simulink model "SOCPIControlBenchmark"  (R2021a)
settings: Solver=FixedStepAuto  StartTime=0.0  StopTime=tsim  FixedStep=0.01  RelTol=1e-3
values from neighbouring files (symbols this model uses):
  ET_Armature_Inductance_RO = 1.2298e-11    [benchmarkPIDStartRealDT.m]
  kio = 0.1    [benchmarkPIDStartRealDT.m]
  kpo = 0.3    [benchmarkPIDStartRealDT.m]
  M_Rotor_Inertia_RO = 1.8747e-13    [benchmarkPIDStartRealDT.m]
  maxKi = 0.3    [benchmarkPIDStartRealDT.m]
  maxKp = 0.5    [benchmarkPIDStartRealDT.m]
  minKi = 0.1    [benchmarkPIDStartRealDT.m]
  minKp = 0.1    [benchmarkPIDStartRealDT.m]
  N = 100    [benchmarkPIDStartRealDT.m]
  optimPeriod = 50    [benchmarkPIDStartRealDT.m]
  OVLim = 2    [benchmarkPIDStartRealDT.m]
  refSignalPeriod = optimPeriod    (= 50)    [benchmarkPIDStartRealDT.m]
  resetThreshold = 0.1    [benchmarkPIDStartRealDT.m]
  TSLim = 6    [benchmarkPIDStartRealDT.m]
libraries: fl_lib x11, nesl_utility x11, ee_lib x8, dspmathops x3, pid_lib x2, simulink x1
(part 2 of 4)

== matlab function SOCPIControlBenchmark/Original NM/Original NM Control/Original NM ==
  data: f input; y output size=2; x input; NM_state_val output
function [y, NM_state_val] = fcn(f, x)
% Acknowledgement goes to Mathworks' FMINSEARCH, borrowed some code snippets
% persistent count

persistent NM_state         %Integer definition for states, since enum is not supported
persistent Full_eval_count
persistent usual_delta      %5 percent deltas for non-zero terms
persistent zero_term_delta  %Even smaller delta for zero elements of x
persistent v fv v_r v_e v_m f_r v_c

n = 2;      %Input dimension - needs to be defined as a constant to keep Simulink port width inheretence happy
np1 = n+1;

n_r = 1/n;  %Calculate reciprocal at compilation time for mean calculation

%Simplex update coefficients %Can be a function of dimension see Han2010
alpha = 1;
beta = 2;
gamma = 0.5;
delta = 0.5;

%Adaptive simplex search coefficients: Han2010
% alpha = 1;
% beta = 1 + 2*n_r;
% gamma = 0.75 - 0.5*n_r;
% delta = 1 - n_r;
% 
% alpha = 0.25;
% beta = 1 + 2*n_r;
% gamma = 0.75 - 0.5*n_r;
% delta = 1 - n_r;


%NM_state:  
    %0 - Initial   (Initialize vertices)+++++
    %1 - FVE: Full vertex evaluation (with insertion sort after each
    %evaluation)++++++
    %2 - Insertion Sort (After Reflection, Expansion or Contraction Steps)
    %3 - Reflection Entry
    %4 - Reflection Evaluate+++++++++++++++++
    %5 - Expansion++++++++++++
    %6 - Outside Contraction++++++++++++
    %7 - Inside Contraction++++++++++++++++
    %(8) - Shrink (Implicit on contraction outcome)

%Full_eval_count:
    %Number of initial vertices evaluated


xin = x(:);         %Force xin to be a column vector

    if isempty(NM_state)
        v = zeros(n,np1);   %Initialize n+1 vertices for simplex
        fv = zeros(1,np1);  %function values at the vertices
        fv(1)=f;%initialize in the initial condition the first vertex
        
        
        v_m = v(:,1);       %0 vector centroid
        v_r = v_m;          %0 vector reflection   
        v_e = v_m;          %0 vector expansion
        v_c = v_m;          %0 vector contraction
        f_r = 0;          %0 vector

        usual_delta = 0.05;
        zero_term_delta = 0.00025;
        NM_state = 0;          %Initial state
        Full_eval_count = 1;   %No vertices evaulated, yet

        v(:,1) = xin;
        for j=1:n
            vt = xin;
            if vt(j) ~= 0
                vt(j) = (1 + usual_delta)*vt(j);
            else
                vt(j) = zero_term_delta;
            end
            v(:, j+1) = vt;
        end
        v;
    end
           
    switch NM_state  
        case 0 %Vertices has just been initialized
          y = v(:, Full_eval_count); %Write out first vertex for evaluation
          NM_state = 1;
          
        case 1 %Full vertex evaluation  and reflection on the final part
            fv(Full_eval_count) = f;  %Read evaluated function value
            
            %sort values
            j = Full_eval_count;  %New value came in, insert it into sorted list
            while ( (j>1) && (fv(j-1)>fv(j)) ) %Sort ascending
               temp = fv(j-1);
               fv(j-1) = fv(j);
               fv(j) = temp;
               temp = v(:, j-1);
               v(:, j-1) = v(:, j); %Also sort corresponding (evaluated) vertices 
               v(:, j) = temp;
               j = j-1;
            end
             
            Full_eval_count = Full_eval_count + 1;            
            if (Full_eval_count <= (np1))
                y = v(:, Full_eval_count);                
            else
                Full_eval_count = Full_eval_count - 1; 
                %NM_state = 3;   %Full vertex evaluation complete -> Reflection 
                v_sum = xin*0;  %Initialize sum for mean calculation

                for i=1:n
                    v_sum = v_sum + v(:, i);
                end

                v_m = v_sum*n_r; %Centroid (mean point of the two best points)
                v_r  = v_m*(1+alpha) - alpha*v(:, end);   %reflection vertex calculation
                y  = v_r;       %set as next output the reflection vertex
                NM_state = 4;   %jump to Reflection Evaluate
            end
            
%         case 2 %Insertion Sort                        
%                 j = Full_eval_count;  %New value came in, insert it into list
%                    while ( (j>1) && (fv(j-1)>fv(j)) ) %Sort ascending
%                        temp = fv(j-1);
%                        fv(j-1) = fv(j);
%                        fv(j) = temp;
%                        temp = v(:, j-1);
%                        v(:, j-1) = v(:, j); %Also sort corresponding (evaluated) vertices 
%                        v(:, j) = temp;
%                        j = j-1;
%                    end
%                 NM_state = 3;   %Reflection 
            
%         case 3 %Reflection Entry
%                 v_sum = xin*0;  %Initialize sum for mean calculation
% 
%                 for i=1:n
%                     v_sum = v_sum + v(:, i);
%                 end
% 
%                 v_m = v_sum*n_r; %Centroid
%                 v_r  = v_m*(1+alpha) - alpha*v(:, np1);
%                 y  = v_r;
%                 NM_state = 4;   %Reflection Evaluate

        case 4 %Reflection Evaluation (after reflection is calculated and applied on the previous step)
            f_r = f;
%             if ( (f_r<fv(:, 1)) && (f_r>fv(:, n)) )  

            if ( (f_r>fv(:, 1)) && (f_r<fv(:, n)) )  
                v(:, np1) = v_r;
                fv(np1) = f_r;
                %NM_state = 2;
                j = Full_eval_count;  %New value came in, insert it into list
                while ( (j>1) && (fv(j-1)>fv(j)) ) %Sort ascending
                   temp = fv(j-1);
                   fv(j-1) = fv(j);
                   fv(j) = temp;
                   temp = v(:, j-1);
                   v(:, j-1) = v(:, j); %Also sort corresponding (evaluated) vertices 
                   v(:, j) = temp;
                   j = j-1;
                end
                %%NM_state = 3;   %Reflection 

                v_sum = xin*0;  %Initialize sum for mean calculation

                for i=1:n
                    v_sum = v_sum + v(:, i);
                end

                v_m = v_sum*n_r; %Centroid
                v_r  = v_m*(1+alpha) - alpha*v(:, np1);
                y  = v_r;
                NM_state = 4;    %Reflection Evaluate
            elseif (f_r<fv(:, 1))
                v_e  = v_m*(1-beta) + beta*v_r; 
                y  = v_e;
                NM_state = 5;    %Expansion
            else
                if ( (f_r>=fv(n)) && (f_r<fv(np1)) ) 
                    v_c  = v_m*(1-gamma) + gamma*v_r; 
                    NM_state = 6; %Outside Contraction
                elseif (f_r>=fv(np1))  
                    v_c  = v_m*(1+gamma) - gamma*v_r; 
                    NM_state = 7; %Inside Contraction
                end
                y = v_c;
            end
            
        case 5 %Expansion
            f_e = f;
            if (f_e<f_r)
                v(:, end) = v_e;
                fv(end) = f_e;
                %NM_state = 2;
                    j = Full_eval_count;  %New value came in, insert it into list
                   while ( (j>1) && (fv(j-1)>fv(j)) ) %Sort ascending
                       temp = fv(j-1);
                       fv(j-1) = fv(j);
                       fv(j) = temp;
                       temp = v(:, j-1);
                       v(:, j-1) = v(:, j); %Also sort corresponding (evaluated) vertices 
                       v(:, j) = temp;
                       j = j-1;
                   end
                %%NM_state = 3;   %Reflection 

                v_sum = xin*0;  %Initialize sum for mean calculation

                for i=1:n
                    v_sum = v_sum + v(:, i);
                end

                v_m = v_sum*n_r; %Centroid
                v_r  = v_m*(1+alpha) - alpha*v(:, np1);
                y  = v_r;
                NM_state = 4;   %Reflection Evaluate
             else
                v(:, np1) = v_r;
                fv(np1) = f_r;
                %NM_state = 2;
                j = Full_eval_count;  %New value came in, insert it into list
               while ( (j>1) && (fv(j-1)>fv(j)) ) %Sort ascending
                   temp = fv(j-1);
                   fv(j-1) = fv(j);
                   fv(j) = temp;
                   temp = v(:, j-1);
                   v(:, j-1) = v(:, j); %Also sort corresponding (evaluated) vertices 
                   v(:, j) = temp;
                   j = j-1;
               end
               
               %%NM_state = 3;   %Reflection 

                v_sum = xin*0;  %Initialize sum for mean calculation

                for i=1:n
                    v_sum = v_sum + v(:, i);
                end

                v_m = v_sum*n_r; %Centroid
                v_r  = v_m*(1+alpha) - alpha*v(:, np1);
                y  = v_r;
                NM_state = 4;   %Reflection Evaluate
            end
            
       case 6 %Contraction
           f_c = f;
           if (f_c<f_r)
               v(:, np1) = v_c;
               fv(np1) = f_c;
               %NM_state = 2;
               j = Full_eval_count;  %New value came in, insert it into list
               while ( (j>1) && (fv(j-1)>fv(j)) ) %Sort ascending
                   temp = fv(j-1);
                   fv(j-1) = fv(j);
                   fv(j) = temp;
                   temp = v(:, j-1);
                   v(:, j-1) = v(:, j); %Also sort corresponding (evaluated) vertices 
                   v(:, j) = temp;
                   j = j-1;
               end
                %%NM_state = 3;   %Reflection 

                v_sum = xin*0;  %Initialize sum for mean calculation

                for i=1:n
                    v_sum = v_sum + v(:, i);
                end

                v_m = v_sum*n_r; %Centroid
                v_r  = v_m*(1+alpha) - alpha*v(:, np1);
                y  = v_r;
                NM_state = 4;   %Reflection Evaluate
           else
               for j=2:n+1   %Shrink
                 v(:,j) = v(:,1)*(1-delta) + delta*v(:,j);
               end
               y = v(:, 2);   %Start with evaluation
               Full_eval_count = 2; 
               NM_state = 1; %Full vertex evaluation after shrink
           end
        case 7
            f_c = f;
               if (f_c<fv(np1))
                   v(:, np1) = v_c;
                   fv(np1) = f_c;
                   %NM_state = 2;
                    j = Full_eval_count;  %New value came in, insert it into list
                    while ( (j>1) && (fv(j-1)>fv(j)) ) %Sort ascending
                       temp = fv(j-1);
                       fv(j-1) = fv(j);
                       fv(j) = temp;
                       temp = v(:, j-1);
                       v(:, j-1) = v(:, j); %Also sort corresponding (evaluated) vertices 
                       v(:, j) = temp;
                       j = j-1;
                    end
                    %%NM_state = 3;   %Reflection 

                    v_sum = xin*0;  %Initialize sum for mean calculation

                    for i=1:n
                        v_sum = v_sum + v(:, i);
                    end

                    v_m = v_sum*n_r; %Centroid
                    v_r  = v_m*(1+alpha) - alpha*v(:, np1);
                    y  = v_r;
                    NM_state = 4;   %Reflection Evaluate
               else
                   for j=2:n+1 %Shrink
                     v(:,j) = v(:,1)*(1-delta) + delta*v(:,j);
                   end
                   y = v(:,2);   %Start with evaluation
                   Full_eval_count = 2; 
                   NM_state = 1; %Full vertex evaluation after shrink  
               end     
        otherwise
        y = v(:,1);
     end %End switch NM_states     
     NM_state_val = NM_state;
end %End of function

== matlab function SOCPIControlBenchmark/Original NM/Original NM Control/Original NM2 ==
  settings: updateMethod=DISCRETE
  data: f input; y output size=2; x input; NM_state_val output
function [y, NM_state_val] = fcn(f, x)
% Acknowledgement goes to Mathworks' FMINSEARCH, borrowed some code snippets
% persistent count

persistent NM_state         %Integer definition for states, since enum is not supported
persistent Full_eval_count
persistent usual_delta      %5 percent deltas for non-zero terms
persistent zero_term_delta  %Even smaller delta for zero elements of x
persistent v fv v_r v_e v_m f_r v_c

n = 2;      %Input dimension - needs to be defined as a constant to keep Simulink port width inheretence happy
np1 = n+1;

n_r = 1/n;  %Calculate reciprocal at compilation time for mean calculation

%Simplex update coefficients %Can be a function of dimension see Han2010
alpha = 1;
beta = 2;
gamma = 0.5;
delta = 0.5;

%Adaptive simplex search coefficients: Han2010
% alpha = 1;
% beta = 1 + 2*n_r;
% gamma = 0.75 - 0.5*n_r;
% delta = 1 - n_r;
% % 
% alpha = 1;           %reflection
% beta = 1 + 2*n_r;       %expansion
% gamma = 0.75 - 0.5*n_r; %contraction
% delta = 1 - n_r;        %shrinking


%NM_state:  
    %0 - Initial   (Initialize vertices)+++++
    %1 - FVE: Full vertex evaluation (with insertion sort after each
    %evaluation)++++++
    %2 - Insertion Sort (After Reflection, Expansion or Contraction Steps)
    %3 - Reflection Entry
    %4 - Reflection Evaluate+++++++++++++++++
    %5 - Expansion++++++++++++
    %6 - Outside Contraction++++++++++++
    %7 - Inside Contraction++++++++++++++++
    %(8) - Shrink (Implicit on contraction outcome)

%Full_eval_count:
    %Number of initial vertices evaluated


xin = x(:);         %Force xin to be a column vector

    if isempty(NM_state)
        v = zeros(n,np1);   %Initialize n+1 vertices for simplex
        fv = zeros(1,np1);  %function values at the vertices
        fv(1)=f;%initialize in the initial condition the first vertex
        
        
        v_m = v(:,1);       %0 vector centroid
        v_r = v_m;          %0 vector reflection   
        v_e = v_m;          %0 vector expansion
        v_c = v_m;          %0 vector contraction
        f_r = 0;          %0 vector

%         usual_delta = 0.05;
        usual_delta = 1;
        zero_term_delta = 0.00025;
        NM_state = 0;          %Initial state
        Full_eval_count = 1;   %No vertices evaulated, yet

        v(:,1) = xin;
        for j=1:n
            vt = xin;
            if vt(j) ~= 0
                vt(j) = (1 + usual_delta)*vt(j);
            else
                vt(j) = zero_term_delta;
            end
            v(:, j+1) = vt;
        end
        v;
    end
           
    switch NM_state  
        case 0 %Vertices has just been initialized
          y = v(:, Full_eval_count); %Write out first vertex for evaluation
          NM_state = 1;
          
        case 1 %Full vertex evaluation  and reflection on the final part
            fv(Full_eval_count) = f;  %Read evaluated function value
            
            %sort values
            j = Full_eval_count;  %New value came in, insert it into sorted list
            while ( (j>1) && (fv(j-1)>fv(j)) ) %Sort ascending
               temp = fv(j-1);
               fv(j-1) = fv(j);
               fv(j) = temp;
               temp = v(:, j-1);
               v(:, j-1) = v(:, j); %Also sort corresponding (evaluated) vertices 
               v(:, j) = temp;
               j = j-1;
            end
             
            Full_eval_count = Full_eval_count + 1;            
            if (Full_eval_count <= (np1))
                y = v(:, Full_eval_count);                
            else
                Full_eval_count = Full_eval_count - 1; 
                %NM_state = 3;   %Full vertex evaluation complete -> Reflection 
                v_sum = xin*0;  %Initialize sum for mean calculation

                for i=1:n
                    v_sum = v_sum + v(:, i);
                end

                v_m = v_sum*n_r; %Centroid (mean point of the two best points)
                v_r  = v_m*(1+alpha) - alpha*v(:, end);   %reflection vertex calculation
                y  = v_r;       %set as next output the reflection vertex
                NM_state = 4;   %jump to Reflection Evaluate
            end
            
%         case 2 %Insertion Sort                        
%                 j = Full_eval_count;  %New value came in, insert it into list
%                    while ( (j>1) && (fv(j-1)>fv(j)) ) %Sort ascending
%                        temp = fv(j-1);
%                        fv(j-1) = fv(j);
%                        fv(j) = temp;
%                        temp = v(:, j-1);
%                        v(:, j-1) = v(:, j); %Also sort corresponding (evaluated) vertices 
%                        v(:, j) = temp;
%                        j = j-1;
%                    end
%                 NM_state = 3;   %Reflection 
            
%         case 3 %Reflection Entry
%                 v_sum = xin*0;  %Initialize sum for mean calculation
% 
%                 for i=1:n
%                     v_sum = v_sum + v(:, i);
%                 end
% 
%                 v_m = v_sum*n_r; %Centroid
%                 v_r  = v_m*(1+alpha) - alpha*v(:, np1);
%                 y  = v_r;
%                 NM_state = 4;   %Reflection Evaluate

        case 4 %Reflection Evaluation (after reflection is calculated and applied on the previous step)
            f_r = f;
%             if ( (f_r<fv(:, 1)) && (f_r>fv(:, n)) )  

            if ( (f_r>fv(:, 1)) && (f_r<fv(:, n)) )  
                v(:, np1) = v_r;
                fv(np1) = f_r;
                %NM_state = 2;
                j = Full_eval_count;  %New value came in, insert it into list
                while ( (j>1) && (fv(j-1)>fv(j)) ) %Sort ascending
                   temp = fv(j-1);
                   fv(j-1) = fv(j);
                   fv(j) = temp;
                   temp = v(:, j-1);
                   v(:, j-1) = v(:, j); %Also sort corresponding (evaluated) vertices 
                   v(:, j) = temp;
                   j = j-1;
                end
                %%NM_state = 3;   %Reflection 

                v_sum = xin*0;  %Initialize sum for mean calculation

                for i=1:n
                    v_sum = v_sum + v(:, i);
                end

                v_m = v_sum*n_r; %Centroid
                v_r  = v_m*(1+alpha) - alpha*v(:, np1);
                y  = v_r;
                NM_state = 4;    %Reflection Evaluate
            elseif (f_r<fv(:, 1))
                v_e  = v_m*(1-beta) + beta*v_r; 
                y  = v_e;
                NM_state = 5;    %Expansion
            else
                if ( (f_r>=fv(n)) && (f_r<fv(np1)) ) 
                    v_c  = v_m*(1-gamma) + gamma*v_r; 
                    NM_state = 6; %Outside Contraction
                elseif (f_r>=fv(np1))  
                    v_c  = v_m*(1+gamma) - gamma*v_r; 
                    NM_state = 7; %Inside Contraction
                end
                y = v_c;
            end
            
        case 5 %Expansion
            f_e = f;
            if (f_e<f_r)
                v(:, end) = v_e;
                fv(end) = f_e;
                %NM_state = 2;
                    j = Full_eval_count;  %New value came in, insert it into list
                   while ( (j>1) && (fv(j-1)>fv(j)) ) %Sort ascending
                       temp = fv(j-1);
                       fv(j-1) = fv(j);
                       fv(j) = temp;
                       temp = v(:, j-1);
                       v(:, j-1) = v(:, j); %Also sort corresponding (evaluated) vertices 
                       v(:, j) = temp;
                       j = j-1;
                   end
                %%NM_state = 3;   %Reflection 

                v_sum = xin*0;  %Initialize sum for mean calculation

                for i=1:n
                    v_sum = v_sum + v(:, i);
                end

                v_m = v_sum*n_r; %Centroid
                v_r  = v_m*(1+alpha) - alpha*v(:, np1);
                y  = v_r;
                NM_state = 4;   %Reflection Evaluate
             else
                v(:, np1) = v_r;
                fv(np1) = f_r;
                %NM_state = 2;
                j = Full_eval_count;  %New value came in, insert it into list
               while ( (j>1) && (fv(j-1)>fv(j)) ) %Sort ascending
                   temp = fv(j-1);
                   fv(j-1) = fv(j);
                   fv(j) = temp;
                   temp = v(:, j-1);
                   v(:, j-1) = v(:, j); %Also sort corresponding (evaluated) vertices 
                   v(:, j) = temp;
                   j = j-1;
               end
               
               %%NM_state = 3;   %Reflection 

                v_sum = xin*0;  %Initialize sum for mean calculation

                for i=1:n
                    v_sum = v_sum + v(:, i);
                end

                v_m = v_sum*n_r; %Centroid
                v_r  = v_m*(1+alpha) - alpha*v(:, np1);
                y  = v_r;
                NM_state = 4;   %Reflection Evaluate
            end
            
       case 6 %Contraction
           f_c = f;
           if (f_c<f_r)
               v(:, np1) = v_c;
               fv(np1) = f_c;
               %NM_state = 2;
               j = Full_eval_count;  %New value came in, insert it into list
               while ( (j>1) && (fv(j-1)>fv(j)) ) %Sort ascending
                   temp = fv(j-1);
                   fv(j-1) = fv(j);
                   fv(j) = temp;
                   temp = v(:, j-1);
                   v(:, j-1) = v(:, j); %Also sort corresponding (evaluated) vertices 
                   v(:, j) = temp;
                   j = j-1;
               end
                %%NM_state = 3;   %Reflection 

                v_sum = xin*0;  %Initialize sum for mean calculation

                for i=1:n
                    v_sum = v_sum + v(:, i);
                end

                v_m = v_sum*n_r; %Centroid
                v_r  = v_m*(1+alpha) - alpha*v(:, np1);
                y  = v_r;
                NM_state = 4;   %Reflection Evaluate
           else
               for j=2:n+1   %Shrink
                 v(:,j) = v(:,1)*(1-delta) + delta*v(:,j);
               end
               y = v(:, 2);   %Start with evaluation
               Full_eval_count = 2; 
               NM_state = 1; %Full vertex evaluation after shrink
           end
        case 7
            f_c = f;
               if (f_c<fv(np1))
                   v(:, np1) = v_c;
                   fv(np1) = f_c;
                   %NM_state = 2;
                    j = Full_eval_count;  %New value came in, insert it into list
                    while ( (j>1) && (fv(j-1)>fv(j)) ) %Sort ascending
                       temp = fv(j-1);
                       fv(j-1) = fv(j);
                       fv(j) = temp;
                       temp = v(:, j-1);
                       v(:, j-1) = v(:, j); %Also sort corresponding (evaluated) vertices 
                       v(:, j) = temp;
                       j = j-1;
                    end
                    %%NM_state = 3;   %Reflection 

                    v_sum = xin*0;  %Initialize sum for mean calculation

                    for i=1:n
                        v_sum = v_sum + v(:, i);
                    end

                    v_m = v_sum*n_r; %Centroid
                    v_r  = v_m*(1+alpha) - alpha*v(:, np1);
                    y  = v_r;
                    NM_state = 4;   %Reflection Evaluate
               else
                   for j=2:n+1 %Shrink
                     v(:,j) = v(:,1)*(1-delta) + delta*v(:,j);
                   end
                   y = v(:,2);   %Start with evaluation
                   Full_eval_count = 2; 
                   NM_state = 1; %Full vertex evaluation after shrink  
               end     
        otherwise
        y = v(:,1);
     end %End switch NM_states     
     NM_state_val = NM_state;
end %End of function

== matlab function SOCPIControlBenchmark/Original NM/Cost function1/MATLAB Function ==
  settings: updateMethod=DISCRETE
  data: y input; tsf output; time input; ovf output; epsilon input; r input; period input; yTotal input; samplingTime input
function [tsf,ovf] = performance(y,time,epsilon,r,period,yTotal,samplingTime)
        persistent OV tsFlag yHist counter ts;
        
        %initialization state
          if isempty(OV)        
              OV=0;
              tsFlag=1;
              yHist=zeros(1,round(period/(2*samplingTime)));
%               ts=0;
              counter=1;
              ts=0*samplingTime;
              tsf=0;
          end
          
          yHist(counter)=yTotal;
          
          %overshoot calculation
          OVCurrent=max(y);
          if OVCurrent>OV
              OV=OVCurrent;
              ovf=OV;
          else
              ovf=OV;
          end
          
          %calculate settling time each half of the period
          if mod(time,round(period/2))==0    
            ts=converTimeInv1s(yHist,10,epsilon);
%             yHist=zeros(1,round(period/2));
            counter=0;
            tsf=ts*samplingTime;
          else
              tsf=ts*samplingTime;
          end
          
          
          if mod(time,period)==0    %restart constraints after each repetitive period
            OV=0;
          end
          
          counter=counter+1;
          
%           
%           if std(y)<epsilon && tsFlag==1 && r==1 %settling time on the low state
%               ts=time;
%               tsFlag=0;
%           else
%               ts=5;
%           end
          

end

== matlab function SOCPIControlBenchmark/GCNM/Cost function2/Cost function ==
  settings: updateMethod=DISCRETE
  data: y input; tsf output; time input; ovf output; epsilon input; r input; period input; yTotal input; samplingTime input; refAmplitude input
function [tsf,ovf] = performance(y,time,epsilon,r,period,yTotal,samplingTime,refAmplitude)
        persistent OV tsFlag yHist counter ts PmAprox;
        
        %initialization state
          if isempty(OV)        
              OV=0;
              PmAprox=0;
              tsFlag=1;
              yHist=zeros(1,round(period/(1*samplingTime)));
%               ts=0;
              counter=1;
              ts=0*samplingTime;
              tsf=0;
          end
          
          yHist(counter)=yTotal;
          
          %overshoot and phase margin calculation 
          OVCurrent=(max(y)-refAmplitude);
          tsFlag=max(y);
          if OVCurrent>OV
              OV=OVCurrent;
              ovf=OV;
              OVPor=abs(OV)/refAmplitude+1e-3;     %overshoot percentage
%               OVPor=abs(OV-refAmplitude+0.001)/refAmplitude;     %overshoot percentage
%               PmAprox= 100*( -log(OVPor)/ sqrt( pi^2+log(OVPor)^2 )); %approximated phase margin (based on second order system approximation)
%               PmAproxf=PmAprox;
          else
              ovf=OV;
              PmAproxf=PmAprox;
          end
          
          %calculate settling time each half of the period
          if mod(time,round(period/2))==0    
            ts=converTimeInv(yHist(1:(end/2)),1,epsilon);
%             ts=converTimeInv(yHist,10,epsilon,refAmplitude);
%             yHist=zeros(1,round(period/2));
            counter=0;
            tsf=ts*samplingTime;
            yHist=zeros(1,round(period/(1*samplingTime)));
          else
              tsf=ts*samplingTime;
          end
          
          
          if mod(time,period)==0    %restart constraints after each repetitive period
            OV=0;
            ts=0;
            PmAprox=0;
            yHist=zeros(1,round(period/(1*samplingTime)));
          end
          
          counter=counter+1;
          

end

== matlab function SOCPIControlBenchmark/Original NM/Cost function/MATLAB Function ==
  settings: updateMethod=DISCRETE
  data: y input; tsf output; time input; ovf output; epsilon input; r input; period input; yTotal input; samplingTime input
function [tsf,ovf] = performance(y,time,epsilon,r,period,yTotal,samplingTime)
        persistent OV tsFlag yHist counter ts;
        
        %initialization state
          if isempty(OV)        
              OV=0;
              tsFlag=1;
              yHist=zeros(1,round(period/(1*samplingTime)));
%               ts=0;
              counter=1;
              ts=0*samplingTime;
              tsf=0;
          end
          
          yHist(counter)=yTotal;
          
          %overshoot calculation
          OVCurrent=max(y);
          if OVCurrent>OV
              OV=OVCurrent;
              ovf=OV;
          else
              ovf=OV;
          end
          
          %calculate settling time each half of the period
          if mod(time,round(period/2))==0    
            ts=converTimeInv1s(yHist(1:round(end/2)),10,epsilon);
%             yHist=zeros(1,round(period/2));
            counter=0;
            tsf=ts*samplingTime;
          else
              tsf=ts*samplingTime;
          end
          
          
          if mod(time,period)==0    %restart constraints after each repetitive period
            OV=0;
          end
          
          counter=counter+1;
          

end
